simulink model "PMSMWithThermal"  (R2024b)
settings: Solver=VariableStepAuto  StartTime=0.0  StopTime=5  RelTol=1e-3  AbsTol=1e-3
PreLoadFcn:
  | PMSMWithThermalParameters;
values from neighbouring files (symbols this model uses):
  B = 0    [param.mat]
  dt = 0.5e-4    (= 5e-05)    [PMSMWithThermalParameters.m]    (also in param.mat)
  dt_speed_control = 0.001    [PMSMWithThermalParameters.m]    (also in param.mat)
  ESO_w0 = 0    [param.mat]
  J = 0.02    [param.mat]
  max_power = 50e3    (= 50000)    [PMSMWithThermalParameters.m]    (also in param.mat)
  max_torque = 220    [PMSMWithThermalParameters.m]    (also in param.mat)
  N = 6    [PMSMWithThermalParameters.m]    (also in param.mat)
  Rs = 0.013    [PMSMWithThermalParameters.m]    (also in param.mat = 1.3)
undefined symbols (not defined in the file or in its folder): DiscIntNeverNeededParam
libraries: fl_lib x124, nesl_utility x33, fl_ps_legacy_lib x3, ee_lib x1, simulink x1
(part 2 of 2)

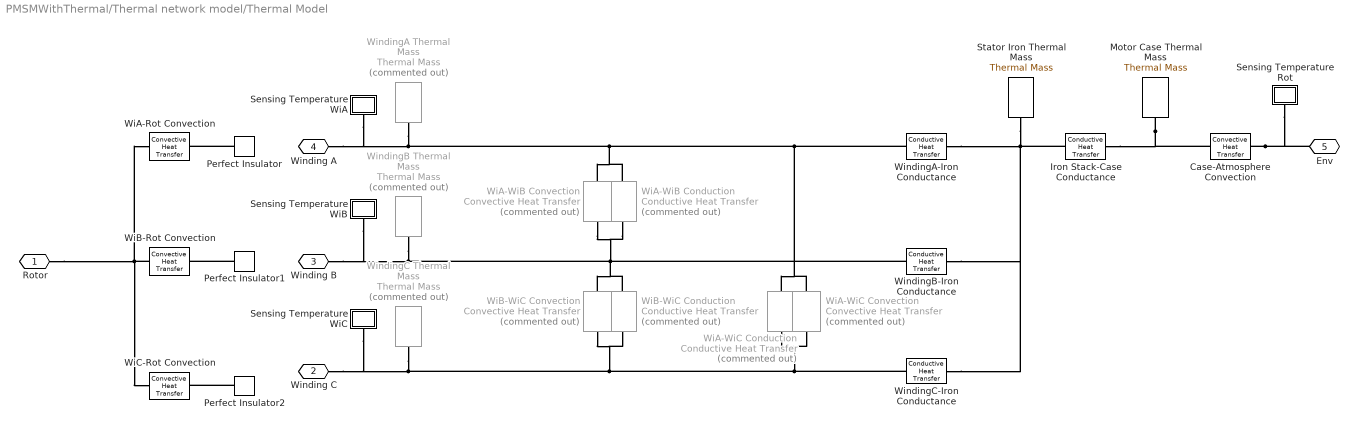
== system PMSMWithThermal/Thermal network model/Thermal Model ==
  Case-Atmosphere Convection : fl_lib/Thermal/Thermal Elements/Convective Heat Transfer  thermal_type=foundation.enum.constant_variable.constant  area=4240 cm^2  heat_tr_coeff=26.8 W/(m^2 * K)  min_heat_tr_coeff=1e-3 W/(K*m^2)  T_specify=off  T_priority=None  T=0 K  T_nominal_specify=off  T_nominal_value=1  T_nominal_unit=K  Q_specify=off  Q_priority=None  Q=0 W  Q_nominal_specify=off  Q_nominal_value=1  Q_nominal_unit=W
  Iron Stack-Case Conductance : fl_lib/Thermal/Thermal Elements/Conductive Heat Transfer  thermal_type=foundation.enum.ConstantVariableTabulated.Constant  wall_geometry=foundation.enum.ConductionWallGeometry.Planar  area=4350 cm^2  thickness=26 cm  d_in=0.05 m  d_out=0.1 m  L=1 m  th_cond_min=10 W/(K*m)  th_cond=80.2 W/(m*K)  th_cond_TLU=[413, 401, 392, 383, 371, 357, 342] W/(K*m)  temp_TLU=[200, 273, 400, 600, 800, 1000, 1200] K  T_specify=off  T_priority=None  T=0 K  T_nominal_specify=off  T_nominal_value=1  T_nominal_unit=K  Q_specify=off  Q_priority=None  Q=0 W  Q_nominal_specify=off  Q_nominal_value=1  Q_nominal_unit=W
  Motor Case Thermal Mass : fl_lib/Thermal/Thermal Elements/Thermal Mass  mass_type=foundation.enum.constant_variable.constant  mass=3.8 kg  sp_heat=903 J/kg/K  mass_min=1e-6 kg  num_ports=foundation.enum.numPorts2.one  m_specify=off  m_priority=High  m=1 kg  m_nominal_specify=off  m_nominal_value=1  m_nominal_unit=kg  T_specify=off  T_priority=High  T=300 K  T_nominal_specify=off  T_nominal_value=1  T_nominal_unit=K  Q_specify=off  Q_priority=None  Q=0 W  Q_nominal_specify=off  Q_nominal_value=1  Q_nominal_unit=W
  Perfect Insulator : fl_lib/Thermal/Thermal Elements/Perfect Insulator  T_specify=off  T_priority=None  T=293.15 K  T_nominal_specify=off  T_nominal_value=1  T_nominal_unit=K
  Perfect Insulator1 : fl_lib/Thermal/Thermal Elements/Perfect Insulator  T_specify=off  T_priority=None  T=293.15 K  T_nominal_specify=off  T_nominal_value=1  T_nominal_unit=K
  Perfect Insulator2 : fl_lib/Thermal/Thermal Elements/Perfect Insulator  T_specify=off  T_priority=None  T=293.15 K  T_nominal_specify=off  T_nominal_value=1  T_nominal_unit=K
  Sensing Temperature Rot : Subsystem
      mask Display: disp('TR')
  Sensing Temperature WiA : Subsystem
      mask Display: disp('TA')
  Sensing Temperature WiB : Subsystem
      mask Display: disp('TB')
  Sensing Temperature WiC : Subsystem
      mask Display: disp('TC')
  Stator Iron Thermal Mass : fl_lib/Thermal/Thermal Elements/Thermal Mass  mass_type=foundation.enum.constant_variable.constant  mass=4.1 kg  sp_heat=447 J/kg/K  mass_min=1e-6 kg  num_ports=foundation.enum.numPorts2.one  m_specify=off  m_priority=High  m=1 kg  m_nominal_specify=off  m_nominal_value=1  m_nominal_unit=kg  T_specify=off  T_priority=High  T=300 K  T_nominal_specify=off  T_nominal_value=1  T_nominal_unit=K  Q_specify=off  Q_priority=None  Q=0 W  Q_nominal_specify=off  Q_nominal_value=1  Q_nominal_unit=W
  WiA-Rot Convection : fl_lib/Thermal/Thermal Elements/Convective Heat Transfer  thermal_type=foundation.enum.constant_variable.constant  area=0.02 m^2  heat_tr_coeff=200 W/(m^2 * K)  min_heat_tr_coeff=1e-3 W/(K*m^2)  T_specify=off  T_priority=None  T=0 K  T_nominal_specify=off  T_nominal_value=1  T_nominal_unit=K  Q_specify=off  Q_priority=None  Q=0 J/s  Q_nominal_specify=off  Q_nominal_value=1  Q_nominal_unit=J/s
  WiA-WiB Conduction : fl_lib/Thermal/Thermal Elements/Conductive Heat Transfer  Commented=on  thermal_type=foundation.enum.ConstantVariableTabulated.Constant  wall_geometry=foundation.enum.ConductionWallGeometry.Planar  area=0.002 m^2  thickness=0.1 m  d_in=0.05 m  d_out=0.1 m  L=1 m  th_cond_min=10 W/(K*m)  th_cond=80 W/(m*K)  th_cond_TLU=[413, 401, 392, 383, 371, 357, 342] W/(K*m)  temp_TLU=[200, 273, 400, 600, 800, 1000, 1200] K  T_specify=off  T_priority=None  T=0 K  T_nominal_specify=off  T_nominal_value=1  T_nominal_unit=K  Q_specify=off  Q_priority=None  Q=0 J/s  Q_nominal_specify=off  Q_nominal_value=1  Q_nominal_unit=J/s
  WiA-WiB Convection : fl_lib/Thermal/Thermal Elements/Convective Heat Transfer  Commented=on  thermal_type=foundation.enum.constant_variable.constant  area=0.004 m^2  heat_tr_coeff=200 W/(m^2 * K)  min_heat_tr_coeff=1e-3 W/(K*m^2)  T_specify=off  T_priority=None  T=0 K  T_nominal_specify=off  T_nominal_value=1  T_nominal_unit=K  Q_specify=off  Q_priority=None  Q=0 J/s  Q_nominal_specify=off  Q_nominal_value=1  Q_nominal_unit=J/s
  WiA-WiC Conduction : fl_lib/Thermal/Thermal Elements/Conductive Heat Transfer  Commented=on  thermal_type=foundation.enum.ConstantVariableTabulated.Constant  wall_geometry=foundation.enum.ConductionWallGeometry.Planar  area=0.002 m^2  thickness=0.1 m  d_in=0.05 m  d_out=0.1 m  L=1 m  th_cond_min=10 W/(K*m)  th_cond=80 W/(m*K)  th_cond_TLU=[413, 401, 392, 383, 371, 357, 342] W/(K*m)  temp_TLU=[200, 273, 400, 600, 800, 1000, 1200] K  T_specify=off  T_priority=None  T=0 K  T_nominal_specify=off  T_nominal_value=1  T_nominal_unit=K  Q_specify=off  Q_priority=None  Q=0 J/s  Q_nominal_specify=off  Q_nominal_value=1  Q_nominal_unit=J/s
  WiA-WiC Convection : fl_lib/Thermal/Thermal Elements/Convective Heat Transfer  Commented=on  thermal_type=foundation.enum.constant_variable.constant  area=0.004 m^2  heat_tr_coeff=200 W/(m^2 * K)  min_heat_tr_coeff=1e-3 W/(K*m^2)  T_specify=off  T_priority=None  T=0 K  T_nominal_specify=off  T_nominal_value=1  T_nominal_unit=K  Q_specify=off  Q_priority=None  Q=0 J/s  Q_nominal_specify=off  Q_nominal_value=1  Q_nominal_unit=J/s
  WiB-Rot Convection : fl_lib/Thermal/Thermal Elements/Convective Heat Transfer  thermal_type=foundation.enum.constant_variable.constant  area=0.02 m^2  heat_tr_coeff=200 W/(m^2 * K)  min_heat_tr_coeff=1e-3 W/(K*m^2)  T_specify=off  T_priority=None  T=0 K  T_nominal_specify=off  T_nominal_value=1  T_nominal_unit=K  Q_specify=off  Q_priority=None  Q=0 J/s  Q_nominal_specify=off  Q_nominal_value=1  Q_nominal_unit=J/s
  WiB-WiC Conduction : fl_lib/Thermal/Thermal Elements/Conductive Heat Transfer  Commented=on  thermal_type=foundation.enum.ConstantVariableTabulated.Constant  wall_geometry=foundation.enum.ConductionWallGeometry.Planar  area=0.002 m^2  thickness=0.1 m  d_in=0.05 m  d_out=0.1 m  L=1 m  th_cond_min=10 W/(K*m)  th_cond=80 W/(m*K)  th_cond_TLU=[413, 401, 392, 383, 371, 357, 342] W/(K*m)  temp_TLU=[200, 273, 400, 600, 800, 1000, 1200] K  T_specify=off  T_priority=None  T=0 K  T_nominal_specify=off  T_nominal_value=1  T_nominal_unit=K  Q_specify=off  Q_priority=None  Q=0 J/s  Q_nominal_specify=off  Q_nominal_value=1  Q_nominal_unit=J/s
  WiB-WiC Convection : fl_lib/Thermal/Thermal Elements/Convective Heat Transfer  Commented=on  thermal_type=foundation.enum.constant_variable.constant  area=0.004 m^2  heat_tr_coeff=200 W/(m^2 * K)  min_heat_tr_coeff=1e-3 W/(K*m^2)  T_specify=off  T_priority=None  T=0 K  T_nominal_specify=off  T_nominal_value=1  T_nominal_unit=K  Q_specify=off  Q_priority=None  Q=0 J/s  Q_nominal_specify=off  Q_nominal_value=1  Q_nominal_unit=J/s
  WiC-Rot Convection : fl_lib/Thermal/Thermal Elements/Convective Heat Transfer  thermal_type=foundation.enum.constant_variable.constant  area=0.02 m^2  heat_tr_coeff=200 W/(m^2 * K)  min_heat_tr_coeff=1e-3 W/(K*m^2)  T_specify=off  T_priority=None  T=0 K  T_nominal_specify=off  T_nominal_value=1  T_nominal_unit=K  Q_specify=off  Q_priority=None  Q=0 J/s  Q_nominal_specify=off  Q_nominal_value=1  Q_nominal_unit=J/s
  WindingA Thermal Mass : fl_lib/Thermal/Thermal Elements/Thermal Mass  Commented=on  mass_type=foundation.enum.constant_variable.constant  mass=6.3 kg  sp_heat=385 J/kg/K  mass_min=1e-6 kg  num_ports=foundation.enum.numPorts2.one  m_specify=off  m_priority=High  m=1 kg  m_nominal_specify=off  m_nominal_value=1  m_nominal_unit=kg  T_specify=off  T_priority=High  T=300 K  T_nominal_specify=off  T_nominal_value=1  T_nominal_unit=K  Q_specify=off  Q_priority=None  Q=0 W  Q_nominal_specify=off  Q_nominal_value=1  Q_nominal_unit=W
  WindingA-Iron Conductance : fl_lib/Thermal/Thermal Elements/Conductive Heat Transfer  thermal_type=foundation.enum.ConstantVariableTabulated.Constant  wall_geometry=foundation.enum.ConductionWallGeometry.Planar  area=250 cm^2  thickness=30 cm  d_in=0.05 m  d_out=0.1 m  L=1 m  th_cond_min=10 W/(K*m)  th_cond=360 W/(m*K)  th_cond_TLU=[413, 401, 392, 383, 371, 357, 342] W/(K*m)  temp_TLU=[200, 273, 400, 600, 800, 1000, 1200] K  T_specify=off  T_priority=None  T=0 K  T_nominal_specify=off  T_nominal_value=1  T_nominal_unit=K  Q_specify=off  Q_priority=None  Q=0 W  Q_nominal_specify=off  Q_nominal_value=1  Q_nominal_unit=W
  WindingB Thermal Mass : fl_lib/Thermal/Thermal Elements/Thermal Mass  Commented=on  mass_type=foundation.enum.constant_variable.constant  mass=6.3 kg  sp_heat=385 J/kg/K  mass_min=1e-6 kg  num_ports=foundation.enum.numPorts2.one  m_specify=off  m_priority=High  m=1 kg  m_nominal_specify=off  m_nominal_value=1  m_nominal_unit=kg  T_specify=off  T_priority=High  T=300 K  T_nominal_specify=off  T_nominal_value=1  T_nominal_unit=K  Q_specify=off  Q_priority=None  Q=0 W  Q_nominal_specify=off  Q_nominal_value=1  Q_nominal_unit=W
  WindingB-Iron Conductance : fl_lib/Thermal/Thermal Elements/Conductive Heat Transfer  thermal_type=foundation.enum.ConstantVariableTabulated.Constant  wall_geometry=foundation.enum.ConductionWallGeometry.Planar  area=250 cm^2  thickness=30 cm  d_in=0.05 m  d_out=0.1 m  L=1 m  th_cond_min=10 W/(K*m)  th_cond=360 W/(m*K)  th_cond_TLU=[413, 401, 392, 383, 371, 357, 342] W/(K*m)  temp_TLU=[200, 273, 400, 600, 800, 1000, 1200] K  T_specify=off  T_priority=None  T=0 K  T_nominal_specify=off  T_nominal_value=1  T_nominal_unit=K  Q_specify=off  Q_priority=None  Q=0 W  Q_nominal_specify=off  Q_nominal_value=1  Q_nominal_unit=W
  WindingC Thermal Mass : fl_lib/Thermal/Thermal Elements/Thermal Mass  Commented=on  mass_type=foundation.enum.constant_variable.constant  mass=6.3 kg  sp_heat=385 J/kg/K  mass_min=1e-6 kg  num_ports=foundation.enum.numPorts2.one  m_specify=off  m_priority=High  m=1 kg  m_nominal_specify=off  m_nominal_value=1  m_nominal_unit=kg  T_specify=off  T_priority=High  T=300 K  T_nominal_specify=off  T_nominal_value=1  T_nominal_unit=K  Q_specify=off  Q_priority=None  Q=0 W  Q_nominal_specify=off  Q_nominal_value=1  Q_nominal_unit=W
  WindingC-Iron Conductance : fl_lib/Thermal/Thermal Elements/Conductive Heat Transfer  thermal_type=foundation.enum.ConstantVariableTabulated.Constant  wall_geometry=foundation.enum.ConductionWallGeometry.Planar  area=250 cm^2  thickness=30 cm  d_in=0.05 m  d_out=0.1 m  L=1 m  th_cond_min=10 W/(K*m)  th_cond=360 W/(m*K)  th_cond_TLU=[413, 401, 392, 383, 371, 357, 342] W/(K*m)  temp_TLU=[200, 273, 400, 600, 800, 1000, 1200] K  T_specify=off  T_priority=None  T=0 K  T_nominal_specify=off  T_nominal_value=1  T_nominal_unit=K  Q_specify=off  Q_priority=None  Q=0 W  Q_nominal_specify=off  Q_nominal_value=1  Q_nominal_unit=W
  Rotor : PMIOPort  Side=Left
  Winding C : PMIOPort  Port=2  Side=Right
  Winding B : PMIOPort  Port=3  Side=Right
  Winding A : PMIOPort  Port=4  Side=Right
  Env : PMIOPort  Port=5  Side=Left
  connections:
  Rotor/RConn1 -- WiA-Rot Convection/LConn1 -- WiB-Rot Convection/LConn1 -- WiC-Rot Convection/LConn1
  WindingA-Iron Conductance/LConn1 -- WiA-WiC Conduction/LConn1 -- WiA-WiC Convection/LConn1 -- WiA-WiB Convection/LConn1 -- WiA-WiB Conduction/LConn1 -- Sensing Temperature WiA/LConn1 -- Winding A/RConn1 -- WindingA Thermal Mass/LConn1
  WindingB-Iron Conductance/LConn1 -- WiA-WiB Convection/RConn1 -- WiA-WiB Conduction/RConn1 -- WiB-WiC Convection/LConn1 -- WiB-WiC Conduction/LConn1 -- Winding B/RConn1 -- Sensing Temperature WiB/LConn1 -- WindingB Thermal Mass/LConn1
  WindingC-Iron Conductance/LConn1 -- Winding C/RConn1 -- Sensing Temperature WiC/LConn1 -- WindingC Thermal Mass/LConn1 -- WiB-WiC Convection/RConn1 -- WiB-WiC Conduction/RConn1 -- WiA-WiC Conduction/RConn1 -- WiA-WiC Convection/RConn1
  Perfect Insulator/LConn1 -- WiA-Rot Convection/RConn1
  Perfect Insulator1/LConn1 -- WiB-Rot Convection/RConn1
  Perfect Insulator2/LConn1 -- WiC-Rot Convection/RConn1
  Motor Case Thermal Mass/LConn1 -- Iron Stack-Case Conductance/RConn1 -- Case-Atmosphere Convection/LConn1
  Stator Iron Thermal Mass/LConn1 -- WindingC-Iron Conductance/RConn1 -- WindingB-Iron Conductance/RConn1 -- WindingA-Iron Conductance/RConn1 -- Iron Stack-Case Conductance/LConn1
  Case-Atmosphere Convection/RConn1 -- Env/RConn1 -- Sensing Temperature Rot/LConn1

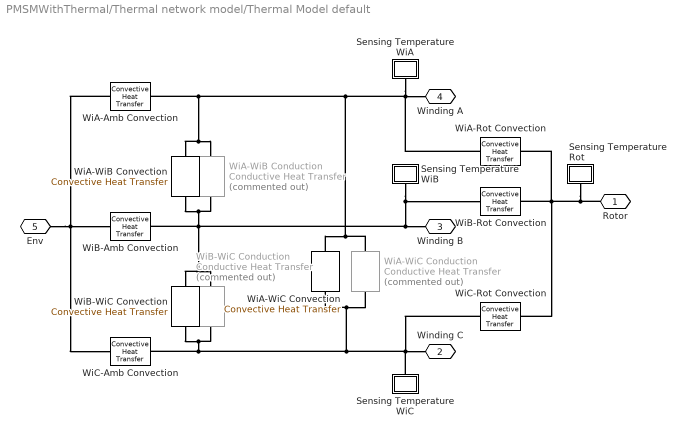
== system PMSMWithThermal/Thermal network model/Thermal Model default ==
  Sensing Temperature Rot : Subsystem
      mask Display: disp('TR')
  Sensing Temperature WiA : Subsystem
      mask Display: disp('TA')
  Sensing Temperature WiB : Subsystem
      mask Display: disp('TB')
  Sensing Temperature WiC : Subsystem
      mask Display: disp('TC')
  WiA-Amb Convection : fl_lib/Thermal/Thermal Elements/Convective Heat Transfer  thermal_type=foundation.enum.constant_variable.constant  area=0.1 m^2  heat_tr_coeff=1 W/(m^2 * K)  min_heat_tr_coeff=1e-3 W/(K*m^2)  T_specify=off  T_priority=None  T=0 K  T_nominal_specify=off  T_nominal_value=1  T_nominal_unit=K  Q_specify=off  Q_priority=None  Q=0 J/s  Q_nominal_specify=off  Q_nominal_value=1  Q_nominal_unit=J/s
  WiA-Rot Convection : fl_lib/Thermal/Thermal Elements/Convective Heat Transfer  thermal_type=foundation.enum.constant_variable.constant  area=0.02 m^2  heat_tr_coeff=200 W/(m^2 * K)  min_heat_tr_coeff=1e-3 W/(K*m^2)  T_specify=off  T_priority=None  T=0 K  T_nominal_specify=off  T_nominal_value=1  T_nominal_unit=K  Q_specify=off  Q_priority=None  Q=0 J/s  Q_nominal_specify=off  Q_nominal_value=1  Q_nominal_unit=J/s
  WiA-WiB Conduction : fl_lib/Thermal/Thermal Elements/Conductive Heat Transfer  Commented=on  thermal_type=foundation.enum.ConstantVariableTabulated.Constant  wall_geometry=foundation.enum.ConductionWallGeometry.Planar  area=0.002 m^2  thickness=0.1 m  d_in=0.05 m  d_out=0.1 m  L=1 m  th_cond_min=10 W/(K*m)  th_cond=80 W/(m*K)  th_cond_TLU=[413, 401, 392, 383, 371, 357, 342] W/(K*m)  temp_TLU=[200, 273, 400, 600, 800, 1000, 1200] K  T_specify=off  T_priority=None  T=0 K  T_nominal_specify=off  T_nominal_value=1  T_nominal_unit=K  Q_specify=off  Q_priority=None  Q=0 J/s  Q_nominal_specify=off  Q_nominal_value=1  Q_nominal_unit=J/s
  WiA-WiB Convection : fl_lib/Thermal/Thermal Elements/Convective Heat Transfer  thermal_type=foundation.enum.constant_variable.constant  area=0.004 m^2  heat_tr_coeff=200 W/(m^2 * K)  min_heat_tr_coeff=1e-3 W/(K*m^2)  T_specify=off  T_priority=None  T=0 K  T_nominal_specify=off  T_nominal_value=1  T_nominal_unit=K  Q_specify=off  Q_priority=None  Q=0 J/s  Q_nominal_specify=off  Q_nominal_value=1  Q_nominal_unit=J/s
  WiA-WiC Conduction : fl_lib/Thermal/Thermal Elements/Conductive Heat Transfer  Commented=on  thermal_type=foundation.enum.ConstantVariableTabulated.Constant  wall_geometry=foundation.enum.ConductionWallGeometry.Planar  area=0.002 m^2  thickness=0.1 m  d_in=0.05 m  d_out=0.1 m  L=1 m  th_cond_min=10 W/(K*m)  th_cond=80 W/(m*K)  th_cond_TLU=[413, 401, 392, 383, 371, 357, 342] W/(K*m)  temp_TLU=[200, 273, 400, 600, 800, 1000, 1200] K  T_specify=off  T_priority=None  T=0 K  T_nominal_specify=off  T_nominal_value=1  T_nominal_unit=K  Q_specify=off  Q_priority=None  Q=0 J/s  Q_nominal_specify=off  Q_nominal_value=1  Q_nominal_unit=J/s
  WiA-WiC Convection : fl_lib/Thermal/Thermal Elements/Convective Heat Transfer  thermal_type=foundation.enum.constant_variable.constant  area=0.004 m^2  heat_tr_coeff=200 W/(m^2 * K)  min_heat_tr_coeff=1e-3 W/(K*m^2)  T_specify=off  T_priority=None  T=0 K  T_nominal_specify=off  T_nominal_value=1  T_nominal_unit=K  Q_specify=off  Q_priority=None  Q=0 J/s  Q_nominal_specify=off  Q_nominal_value=1  Q_nominal_unit=J/s
  WiB-Amb Convection : fl_lib/Thermal/Thermal Elements/Convective Heat Transfer  thermal_type=foundation.enum.constant_variable.constant  area=0.1 m^2  heat_tr_coeff=1 W/(m^2 * K)  min_heat_tr_coeff=1e-3 W/(K*m^2)  T_specify=off  T_priority=None  T=0 K  T_nominal_specify=off  T_nominal_value=1  T_nominal_unit=K  Q_specify=off  Q_priority=None  Q=0 J/s  Q_nominal_specify=off  Q_nominal_value=1  Q_nominal_unit=J/s
  WiB-Rot Convection : fl_lib/Thermal/Thermal Elements/Convective Heat Transfer  thermal_type=foundation.enum.constant_variable.constant  area=0.02 m^2  heat_tr_coeff=200 W/(m^2 * K)  min_heat_tr_coeff=1e-3 W/(K*m^2)  T_specify=off  T_priority=None  T=0 K  T_nominal_specify=off  T_nominal_value=1  T_nominal_unit=K  Q_specify=off  Q_priority=None  Q=0 J/s  Q_nominal_specify=off  Q_nominal_value=1  Q_nominal_unit=J/s
  WiB-WiC Conduction : fl_lib/Thermal/Thermal Elements/Conductive Heat Transfer  Commented=on  thermal_type=foundation.enum.ConstantVariableTabulated.Constant  wall_geometry=foundation.enum.ConductionWallGeometry.Planar  area=0.002 m^2  thickness=0.1 m  d_in=0.05 m  d_out=0.1 m  L=1 m  th_cond_min=10 W/(K*m)  th_cond=80 W/(m*K)  th_cond_TLU=[413, 401, 392, 383, 371, 357, 342] W/(K*m)  temp_TLU=[200, 273, 400, 600, 800, 1000, 1200] K  T_specify=off  T_priority=None  T=0 K  T_nominal_specify=off  T_nominal_value=1  T_nominal_unit=K  Q_specify=off  Q_priority=None  Q=0 J/s  Q_nominal_specify=off  Q_nominal_value=1  Q_nominal_unit=J/s
  WiB-WiC Convection : fl_lib/Thermal/Thermal Elements/Convective Heat Transfer  thermal_type=foundation.enum.constant_variable.constant  area=0.004 m^2  heat_tr_coeff=200 W/(m^2 * K)  min_heat_tr_coeff=1e-3 W/(K*m^2)  T_specify=off  T_priority=None  T=0 K  T_nominal_specify=off  T_nominal_value=1  T_nominal_unit=K  Q_specify=off  Q_priority=None  Q=0 J/s  Q_nominal_specify=off  Q_nominal_value=1  Q_nominal_unit=J/s
  WiC-Amb Convection : fl_lib/Thermal/Thermal Elements/Convective Heat Transfer  thermal_type=foundation.enum.constant_variable.constant  area=0.1 m^2  heat_tr_coeff=1 W/(m^2 * K)  min_heat_tr_coeff=1e-3 W/(K*m^2)  T_specify=off  T_priority=None  T=0 K  T_nominal_specify=off  T_nominal_value=1  T_nominal_unit=K  Q_specify=off  Q_priority=None  Q=0 J/s  Q_nominal_specify=off  Q_nominal_value=1  Q_nominal_unit=J/s
  WiC-Rot Convection : fl_lib/Thermal/Thermal Elements/Convective Heat Transfer  thermal_type=foundation.enum.constant_variable.constant  area=0.02 m^2  heat_tr_coeff=200 W/(m^2 * K)  min_heat_tr_coeff=1e-3 W/(K*m^2)  T_specify=off  T_priority=None  T=0 K  T_nominal_specify=off  T_nominal_value=1  T_nominal_unit=K  Q_specify=off  Q_priority=None  Q=0 J/s  Q_nominal_specify=off  Q_nominal_value=1  Q_nominal_unit=J/s
  Rotor : PMIOPort  Side=Left
  Winding C : PMIOPort  Port=2  Side=Right
  Winding B : PMIOPort  Port=3  Side=Right
  Winding A : PMIOPort  Port=4  Side=Right
  Env : PMIOPort  Port=5  Side=Left
  connections:
  WiA-Rot Convection/RConn1 -- WiA-WiC Conduction/RConn1 -- WiA-WiC Convection/RConn1 -- WiA-WiB Convection/LConn1 -- WiA-WiB Conduction/LConn1 -- WiA-Amb Convection/LConn1 -- Sensing Temperature WiA/LConn1 -- Winding A/RConn1
  Rotor/RConn1 -- Sensing Temperature Rot/LConn1 -- WiC-Rot Convection/LConn1 -- WiB-Rot Convection/LConn1 -- WiA-Rot Convection/LConn1
  WiA-WiB Convection/RConn1 -- WiA-WiB Conduction/RConn1 -- Sensing Temperature WiB/LConn1 -- WiB-Rot Convection/RConn1 -- Winding B/RConn1 -- WiB-Amb Convection/LConn1 -- WiB-WiC Conduction/LConn1 -- WiB-WiC Convection/LConn1
  WiC-Rot Convection/RConn1 -- Winding C/RConn1 -- WiB-WiC Conduction/RConn1 -- WiB-WiC Convection/RConn1 -- WiC-Amb Convection/LConn1 -- WiA-WiC Convection/LConn1 -- WiA-WiC Conduction/LConn1 -- Sensing Temperature WiC/LConn1
  WiA-Amb Convection/RConn1 -- Env/RConn1 -- WiC-Amb Convection/RConn1 -- WiB-Amb Convection/RConn1

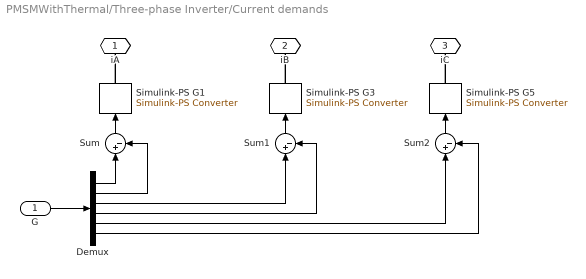
== system PMSMWithThermal/Three-phase Inverter/Current demands ==
  G : Inport
  Demux : Demux  Outputs=[1,1,1,1,1,1]
  Simulink-PS G1 : nesl_utility/Simulink-PS Converter  PhysicalDomain=network_engine_domain  SubClassName=ps_input  LeftPortType=input  RightPortType=output  PseudoPeriodic=off  Frequencies=[]  NoiseDistribution=none  NoiseParameters=[]  Unit=1  AffineConversion=off  FilteringAndDerivatives=zero  SimscapeFilterOrder=1  InputFilterTimeConstant=1e-6  UdotUserProvided=1
  Simulink-PS G3 : nesl_utility/Simulink-PS Converter  PhysicalDomain=network_engine_domain  SubClassName=ps_input  LeftPortType=input  RightPortType=output  PseudoPeriodic=off  Frequencies=[]  NoiseDistribution=none  NoiseParameters=[]  Unit=1  AffineConversion=off  FilteringAndDerivatives=zero  SimscapeFilterOrder=1  InputFilterTimeConstant=1e-6  UdotUserProvided=0
  Simulink-PS G5 : nesl_utility/Simulink-PS Converter  PhysicalDomain=network_engine_domain  SubClassName=ps_input  LeftPortType=input  RightPortType=output  PseudoPeriodic=off  Frequencies=[]  NoiseDistribution=none  NoiseParameters=[]  Unit=1  AffineConversion=off  FilteringAndDerivatives=zero  SimscapeFilterOrder=1  InputFilterTimeConstant=1e-6  UdotUserProvided=0
  Sum : Sum  Inputs=|+-  InputSameDT=on  SaturateOnIntegerOverflow=on  OutDataTypeStr=Inherit: Same as first input
  Sum1 : Sum  Inputs=|+-  InputSameDT=on  SaturateOnIntegerOverflow=on  OutDataTypeStr=Inherit: Same as first input
  Sum2 : Sum  Inputs=|+-  InputSameDT=on  SaturateOnIntegerOverflow=on  OutDataTypeStr=Inherit: Same as first input
  iA : PMIOPort  Side=Right
  iB : PMIOPort  Port=2  Side=Right
  iC : PMIOPort  Port=3  Side=Right
  wires:
  G/1 -> Demux/1
  Demux/4 -> Sum1/2
  Demux/3 -> Sum1/1
  Demux/6 -> Sum2/2
  Sum1/1 -> Simulink-PS G3/1
  Demux/2 -> Sum/2
  Demux/5 -> Sum2/1
  Sum2/1 -> Simulink-PS G5/1
  Sum/1 -> Simulink-PS G1/1
  Demux/1 -> Sum/1
  connections:
  Simulink-PS G1/RConn1 -- iA/RConn1
  Simulink-PS G5/RConn1 -- iC/RConn1
  Simulink-PS G3/RConn1 -- iB/RConn1

== system PMSMWithThermal/Three-phase Inverter/iA ==
  ERef : fl_lib/Electrical/Electrical Elements/Electrical Reference
  PS Product : fl_ps_legacy_lib/Legacy Physical Signals/Functions/PS Product
  Resistor : fl_lib/Electrical/Electrical Elements/Resistor  R=1000 Ohm  i_specify=off  i_priority=High  i=0 A  i_nominal_specify=off  i_nominal_value=1  i_nominal_unit=A  v_specify=off  v_priority=High  v=0 V  v_nominal_specify=off  v_nominal_value=1  v_nominal_unit=V
  Voltage Sensor : fl_lib/Electrical/Electrical Sensors/Voltage Sensor
  iA : fl_lib/Electrical/Electrical Sources/Controlled Current Source
  + : PMIOPort  Side=Right
  P : PMIOPort  Port=2  Side=Right
  ref : PMIOPort  Port=3  Side=Left
  connections:
  iA/LConn1 -- +/RConn1 -- Resistor/RConn1 -- Voltage Sensor/LConn1
  Voltage Sensor/RConn1 -- PS Product/LConn1
  PS Product/RConn1 -- P/RConn1
  ERef/LConn1 -- Resistor/LConn1 -- Voltage Sensor/RConn2 -- iA/RConn2
  iA/RConn1 -- PS Product/LConn2 -- ref/RConn1

== system PMSMWithThermal/Three-phase Inverter/iB ==
  ERef : fl_lib/Electrical/Electrical Elements/Electrical Reference
  PS Product : fl_ps_legacy_lib/Legacy Physical Signals/Functions/PS Product
  Resistor : fl_lib/Electrical/Electrical Elements/Resistor  R=1000 Ohm  i_specify=off  i_priority=High  i=0 A  i_nominal_specify=off  i_nominal_value=1  i_nominal_unit=A  v_specify=off  v_priority=High  v=0 V  v_nominal_specify=off  v_nominal_value=1  v_nominal_unit=V
  Voltage Sensor : fl_lib/Electrical/Electrical Sensors/Voltage Sensor
  iA : fl_lib/Electrical/Electrical Sources/Controlled Current Source
  + : PMIOPort  Side=Right
  P : PMIOPort  Port=2  Side=Right
  ref : PMIOPort  Port=3  Side=Left
  connections:
  ref/RConn1 -- PS Product/LConn2 -- iA/RConn1
  Resistor/LConn1 -- Voltage Sensor/RConn2 -- iA/RConn2 -- ERef/LConn1
  PS Product/RConn1 -- P/RConn1
  Voltage Sensor/RConn1 -- PS Product/LConn1
  +/RConn1 -- Voltage Sensor/LConn1 -- Resistor/RConn1 -- iA/LConn1

== system PMSMWithThermal/Three-phase Inverter/iC ==
  ERef : fl_lib/Electrical/Electrical Elements/Electrical Reference
  PS Product : fl_ps_legacy_lib/Legacy Physical Signals/Functions/PS Product
  Resistor : fl_lib/Electrical/Electrical Elements/Resistor  R=1000 Ohm  i_specify=off  i_priority=High  i=0 A  i_nominal_specify=off  i_nominal_value=1  i_nominal_unit=A  v_specify=off  v_priority=High  v=0 V  v_nominal_specify=off  v_nominal_value=1  v_nominal_unit=V
  Voltage Sensor : fl_lib/Electrical/Electrical Sensors/Voltage Sensor
  iA : fl_lib/Electrical/Electrical Sources/Controlled Current Source
  + : PMIOPort  Side=Right
  P : PMIOPort  Port=2  Side=Right
  ref : PMIOPort  Port=3  Side=Left
  connections:
  iA/LConn1 -- Resistor/RConn1 -- Voltage Sensor/LConn1 -- +/RConn1
  Voltage Sensor/RConn1 -- PS Product/LConn1
  PS Product/RConn1 -- P/RConn1
  ERef/LConn1 -- iA/RConn2 -- Voltage Sensor/RConn2 -- Resistor/LConn1
  iA/RConn1 -- PS Product/LConn2 -- ref/RConn1

== system PMSMWithThermal/PMSM Controller/Vector controller/Current control and gate assignment (averaged) ==
  iRefABC : Inport
  iABC : Inport  Port=2
  Controlled current source assignments : Subsystem
  Terminator : Terminator
  G : Outport  VectorParamsAs1DForOutWhenUnconnected=off
  wires:
  Controlled current source assignments/1(G) -> G/1
  iABC/1 -> Terminator/1
  iRefABC/1 -> Controlled current source assignments/1(iRefABC)

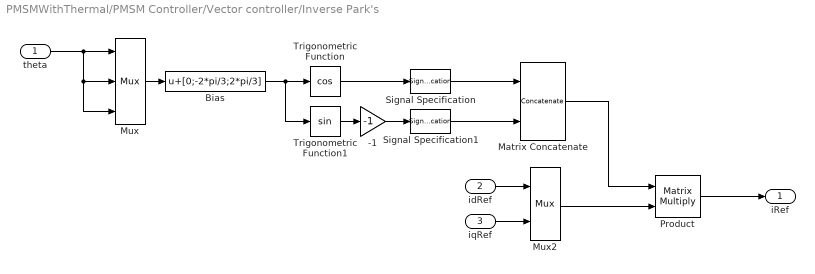
== system PMSMWithThermal/PMSM Controller/Vector controller/Inverse Park's ==
  theta : Inport
  idRef : Inport  Port=2
  iqRef : Inport  Port=3
  -1 : Gain  Gain=-1  SaturateOnIntegerOverflow=on  OutDataTypeStr=Inherit: Same as input  ParamDataTypeStr=Inherit: Same as input
  Bias : Bias  Bias=[0;-2*pi/3;2*pi/3]  SaturateOnIntegerOverflow=off
  Matrix Concatenate : Concatenate  Mode=Multidimensional array  ConcatenateDimension=2
  Mux : Mux  Inputs=3
  Mux2 : Mux  Inputs=2
  Product : Product  Multiplication=Matrix(*)  RndMeth=Zero
  Signal Specification : SignalSpecification  Dimensions=[3 1]
  Signal Specification1 : SignalSpecification  Dimensions=[3 1]
  Trigonometric Function : Trigonometry  Operator=cos
  Trigonometric Function1 : Trigonometry
  iRef : Outport  VectorParamsAs1DForOutWhenUnconnected=off
  wires:
  -1/1 -> Signal Specification1/1
  Trigonometric Function/1 -> Signal Specification/1
  Product/1 -> iRef/1
  theta/1 -> Mux/2, Mux/3, Mux/1
  Bias/1 -> Trigonometric Function1/1, Trigonometric Function/1
  Trigonometric Function1/1 -> -1/1
  Signal Specification1/1 -> Matrix Concatenate/2
  Signal Specification/1 -> Matrix Concatenate/1
  idRef/1 -> Mux2/1
  iqRef/1 -> Mux2/2
  Mux2/1 -> Product/2
  Matrix Concatenate/1 -> Product/1
  Mux/1 -> Bias/1

== system PMSMWithThermal/Speed Controller/Speed controller/Speed controller ==
  wRef : Inport
  wMeas : Inport  Port=2
  Add : Sum  Inputs=|+-
  Add1 : Sum
  Discrete-Time Integrator : DiscreteIntegrator  gainval=Ki  SampleTime=ts  LimitOutput=on  UpperSaturationLimit=trqMax  LowerSaturationLimit=-trqMax  ICPrevOutput=DiscIntNeverNeededParam  ICPrevScaledInput=DiscIntNeverNeededParam
  Kp : Gain  Gain=Kp
  trqRef : Outport  VectorParamsAs1DForOutWhenUnconnected=off
  wires:
  Add/1 -> Discrete-Time Integrator/1, Kp/1
  wMeas/1 -> Add/2
  Discrete-Time Integrator/1 -> Add1/2
  Kp/1 -> Add1/1
  wRef/1 -> Add/1
  Add1/1 -> trqRef/1

== system PMSMWithThermal/Thermal network model/Thermal Model/Sensing Temperature Rot ==
  PS-Simulink Converter : nesl_utility/PS-Simulink Converter  PhysicalDomain=network_engine_domain  SubClassName=ps_output  LeftPortType=input  RightPortType=output  PseudoPeriodic=off  Frequencies=[]  VectorFormat=1-D array  Unit=degC  AffineConversion=on
  Temperature Sensor : fl_lib/Thermal/Thermal Sensors/Temperature Sensor  temperature_measure=foundation.enum.MeasurementReference.difference
  ThRef : fl_lib/Thermal/Thermal Elements/Thermal Reference
  H : PMIOPort  Side=Left
  tag scope: TR=global
  wires:
  PS-Simulink Converter/1 -> [TR]
  connections:
  Temperature Sensor/RConn2 -- PS-Simulink Converter/LConn1
  ThRef/LConn1 -- Temperature Sensor/RConn1
  H/RConn1 -- Temperature Sensor/LConn1

== system PMSMWithThermal/Thermal network model/Thermal Model/Sensing Temperature WiA ==
  PS-Simulink Converter : nesl_utility/PS-Simulink Converter  PhysicalDomain=network_engine_domain  SubClassName=ps_output  LeftPortType=input  RightPortType=output  PseudoPeriodic=off  Frequencies=[]  VectorFormat=1-D array  Unit=degC  AffineConversion=on
  Temperature Sensor : fl_lib/Thermal/Thermal Sensors/Temperature Sensor  temperature_measure=foundation.enum.MeasurementReference.difference
  ThRef : fl_lib/Thermal/Thermal Elements/Thermal Reference
  H : PMIOPort  Side=Left
  tag scope: TA=global
  wires:
  PS-Simulink Converter/1 -> [TA]
  connections:
  H/RConn1 -- Temperature Sensor/LConn1
  ThRef/LConn1 -- Temperature Sensor/RConn1
  Temperature Sensor/RConn2 -- PS-Simulink Converter/LConn1

== system PMSMWithThermal/Thermal network model/Thermal Model/Sensing Temperature WiB ==
  PS-Simulink Converter : nesl_utility/PS-Simulink Converter  PhysicalDomain=network_engine_domain  SubClassName=ps_output  LeftPortType=input  RightPortType=output  PseudoPeriodic=off  Frequencies=[]  VectorFormat=1-D array  Unit=degC  AffineConversion=on
  Temperature Sensor : fl_lib/Thermal/Thermal Sensors/Temperature Sensor  temperature_measure=foundation.enum.MeasurementReference.difference
  ThRef : fl_lib/Thermal/Thermal Elements/Thermal Reference
  H : PMIOPort  Side=Left
  tag scope: TB=global
  wires:
  PS-Simulink Converter/1 -> [TB]
  connections:
  Temperature Sensor/RConn2 -- PS-Simulink Converter/LConn1
  ThRef/LConn1 -- Temperature Sensor/RConn1
  H/RConn1 -- Temperature Sensor/LConn1

== system PMSMWithThermal/Thermal network model/Thermal Model/Sensing Temperature WiC ==
  PS-Simulink Converter : nesl_utility/PS-Simulink Converter  PhysicalDomain=network_engine_domain  SubClassName=ps_output  LeftPortType=input  RightPortType=output  PseudoPeriodic=off  Frequencies=[]  VectorFormat=1-D array  Unit=degC  AffineConversion=on
  Temperature Sensor : fl_lib/Thermal/Thermal Sensors/Temperature Sensor  temperature_measure=foundation.enum.MeasurementReference.difference
  ThRef : fl_lib/Thermal/Thermal Elements/Thermal Reference
  H : PMIOPort  Side=Left
  tag scope: TC=global
  wires:
  PS-Simulink Converter/1 -> [TC]
  connections:
  H/RConn1 -- Temperature Sensor/LConn1
  ThRef/LConn1 -- Temperature Sensor/RConn1
  Temperature Sensor/RConn2 -- PS-Simulink Converter/LConn1

== system PMSMWithThermal/Thermal network model/Thermal Model default/Sensing Temperature Rot ==
  PS-Simulink Converter : nesl_utility/PS-Simulink Converter  PhysicalDomain=network_engine_domain  SubClassName=ps_output  LeftPortType=input  RightPortType=output  PseudoPeriodic=off  Frequencies=[]  VectorFormat=1-D array  Unit=degC  AffineConversion=on
  Temperature Sensor : fl_lib/Thermal/Thermal Sensors/Temperature Sensor  temperature_measure=foundation.enum.MeasurementReference.difference
  ThRef : fl_lib/Thermal/Thermal Elements/Thermal Reference
  H : PMIOPort  Side=Left
  tag scope: TR=global
  wires:
  PS-Simulink Converter/1 -> [TR]
  connections:
  Temperature Sensor/RConn2 -- PS-Simulink Converter/LConn1
  ThRef/LConn1 -- Temperature Sensor/RConn1
  H/RConn1 -- Temperature Sensor/LConn1

== system PMSMWithThermal/Thermal network model/Thermal Model default/Sensing Temperature WiA ==
  PS-Simulink Converter : nesl_utility/PS-Simulink Converter  PhysicalDomain=network_engine_domain  SubClassName=ps_output  LeftPortType=input  RightPortType=output  PseudoPeriodic=off  Frequencies=[]  VectorFormat=1-D array  Unit=degC  AffineConversion=on
  Temperature Sensor : fl_lib/Thermal/Thermal Sensors/Temperature Sensor  temperature_measure=foundation.enum.MeasurementReference.difference
  ThRef : fl_lib/Thermal/Thermal Elements/Thermal Reference
  H : PMIOPort  Side=Left
  tag scope: TA=global
  wires:
  PS-Simulink Converter/1 -> [TA]
  connections:
  H/RConn1 -- Temperature Sensor/LConn1
  ThRef/LConn1 -- Temperature Sensor/RConn1
  Temperature Sensor/RConn2 -- PS-Simulink Converter/LConn1

== system PMSMWithThermal/Thermal network model/Thermal Model default/Sensing Temperature WiB ==
  PS-Simulink Converter : nesl_utility/PS-Simulink Converter  PhysicalDomain=network_engine_domain  SubClassName=ps_output  LeftPortType=input  RightPortType=output  PseudoPeriodic=off  Frequencies=[]  VectorFormat=1-D array  Unit=degC  AffineConversion=on
  Temperature Sensor : fl_lib/Thermal/Thermal Sensors/Temperature Sensor  temperature_measure=foundation.enum.MeasurementReference.difference
  ThRef : fl_lib/Thermal/Thermal Elements/Thermal Reference
  H : PMIOPort  Side=Left
  tag scope: TB=global
  wires:
  PS-Simulink Converter/1 -> [TB]
  connections:
  Temperature Sensor/RConn2 -- PS-Simulink Converter/LConn1
  ThRef/LConn1 -- Temperature Sensor/RConn1
  H/RConn1 -- Temperature Sensor/LConn1

== system PMSMWithThermal/Thermal network model/Thermal Model default/Sensing Temperature WiC ==
  PS-Simulink Converter : nesl_utility/PS-Simulink Converter  PhysicalDomain=network_engine_domain  SubClassName=ps_output  LeftPortType=input  RightPortType=output  PseudoPeriodic=off  Frequencies=[]  VectorFormat=1-D array  Unit=degC  AffineConversion=on
  Temperature Sensor : fl_lib/Thermal/Thermal Sensors/Temperature Sensor  temperature_measure=foundation.enum.MeasurementReference.difference
  ThRef : fl_lib/Thermal/Thermal Elements/Thermal Reference
  H : PMIOPort  Side=Left
  tag scope: TC=global
  wires:
  PS-Simulink Converter/1 -> [TC]
  connections:
  H/RConn1 -- Temperature Sensor/LConn1
  ThRef/LConn1 -- Temperature Sensor/RConn1
  Temperature Sensor/RConn2 -- PS-Simulink Converter/LConn1

== system PMSMWithThermal/PMSM Controller/Vector controller/Current control and gate assignment (averaged)/Controlled current source assignments ==
  iRefABC : Inport
  Constant : Constant  Value=[0;0;0]
  Constant1 : Constant  Value=[0;0;0]
  Demux : Demux  Outputs=3
  Demux1 : Demux  Outputs=3
  Gain : Gain  Gain=-1
  Mux : Mux  Inputs=6
  Switch : Switch  Criteria=u2 > Threshold  SaturateOnIntegerOverflow=off  InputSameDT=off
  Switch1 : Switch  Criteria=u2 > Threshold  SaturateOnIntegerOverflow=off  InputSameDT=off
  G : Outport  VectorParamsAs1DForOutWhenUnconnected=off
  wires:
  Demux1/1 -> Mux/2  "A(low)"
  Demux1/2 -> Mux/4  "B(low)"
  Demux/2 -> Mux/3  "B(high)"
  Demux/1 -> Mux/1  "A(high)"
  iRefABC/1 -> Switch/1, Switch/2, Gain/1
  Mux/1 -> G/1
  Demux1/3 -> Mux/6  "C(low)"
  Demux/3 -> Mux/5  "C(high)"
  Switch/1 -> Demux/1
  Switch1/1 -> Demux1/1
  Gain/1 -> Switch1/1, Switch1/2
  Constant/1 -> Switch/3
  Constant1/1 -> Switch1/3

== matlab function PMSMWithThermal/ESO/MATLAB Function ==
  data: u input; z_hat output; y input; z_prev input; Ae input; Be input; C input; L input; Ts input; d_hat output
function [z_hat, d_hat] = ESO_speed(u, y, z_prev, Ae, Be, C, L, Ts)
% u      : トルク入力（Iq_ref から換算した T_e）
% y      : 観測速度 [rad/s]
% z_prev : 前回の推定状態 [omega_hat; d_hat]
% Ae,Be,C: 拡張系行列
% L      : ESOゲイン（2x1）
% Ts     : サンプリング周期

% 推定誤差
e = y - C * z_prev;

% ESO の連続時間微分
dz = Ae * z_prev + Be * u + L * e;

% オイラー離散化
z_hat = z_prev + Ts * dz;

% 外乱推定値
d_hat = z_hat(2);

== matlab function PMSMWithThermal/cogging_torque/MATLAB Function ==
  data: theta_e input; T output
function T = cogging_torque(theta_e)
    % theta_e: electrical angle [rad]

    A1 = 0.2;   % 1st harmonic amplitude [Nm]
    A2 = 0.05;  % 2nd harmonic
    A3 = 0.02;  % 3rd harmonic

    T = A1*sin(36*theta_e) + A2*sin(72*theta_e) + A3*sin(108*theta_e);
end
